simulink model "altit"  (Simulink 5.0)
settings: Solver=ode23  SolverMode=SingleTasking  StartTime=0.0  StopTime=300  RelTol=1e-3  AbsTol=1e-6
values from neighbouring files (symbols this model uses):
  A = [Xu/m Xw/m 0 -g*cos(theta0) 0;[Zu Zw Zq+m*U0 -m*g*sin(theta0)]/(m-Zwd) 0 ... (first row only)    [altit_simul.m]    (also in lecture11.m = [Yv/m Yp/m (Yr/m-U0) g*cos(theta0); lecture4.m = [Xu/m Xw/m 0 -g*cos(theta0);[Zu Zw Zq+m*U0 -m*g*sin(theta0)])
  B = [Xde/m Xdp/m;Zde/(m-Zwd) Zdp/(m-Zwd);(Mde+Zde*Mwd/(m-Zwd))/Iyy    (Mdp+Zdp*Mwd/(m-Zwd))/Iyy;0 0;0 0]    [altit_simul.m]    (also in lecture11.m = [1/m 0 0;0 1/Ixxp Ixzp;0 Ixzp 1/Izzp;0 0 0]*[Yda Ydr;Lda Ldr; lecture4.m = [Xde/m Xdp/m;Zde/(m-Zwd) Zdp/(m-Zwd);(Mde+Zde*Mwd/(m-Zwd))/I)
  C = [eye(5);zeros(2,5)]    [altit_simul.m]    (also in hw7_1_6243_2003.m = [0 1 r]/[x0 B A*x0]; lecture11.m = [eye(4)]; lecture4.m = [eye(4,4);0 -1/U0 0 1])
  D = [zeros(5,2);[eye(2)]]    [altit_simul.m]    (also in lecture11.m = V; lecture4.m = V)
  JDe = [tau_e 1]    [altit_simul.m]
  JDt = [tau_t 1]    [altit_simul.m]
  JNe = 1    [altit_simul.m]
  JNt = 1    [altit_simul.m]
  K_h = -1*.00116    (= -0.00116)    [altit_simul.m]
  K_q = 1.95*K_th    (= 1.95)    [altit_simul.m]
  K_th = 1    [altit_simul.m]
  K_u = .1    (= 0.1)    [altit_simul.m]
  Khd = [1/(8*abs(tt(ii))) 1]    [altit_simul.m]
  Khn = [1/abs(tt(ii)) 1]    [altit_simul.m]
  Kud = [1/(0.2857*5) 1]    [altit_simul.m]
  Kun = [1/0.2857 1]    [altit_simul.m]
undefined symbols (not defined in the file or in its folder): sigbuilder_block
libraries: simulink x1
settings Model: LastModifiedBy=jonathan How  LimitDataPoints=off  BooleanDataType=off

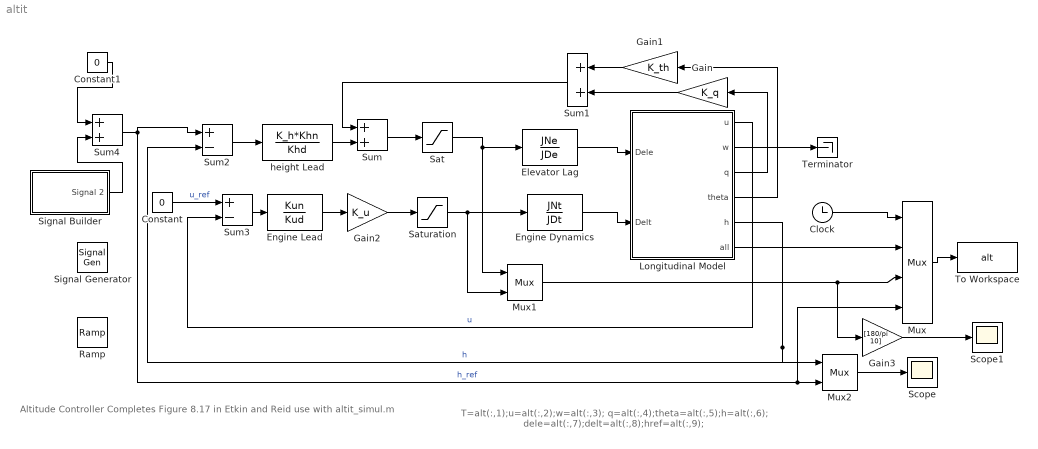
== system altit ==
  note: Altitude Controller
      | Completes Figure 8.17 in Etkin and Reid
      | use with altit_simul.m
  note: T=alt(:,1);u=alt(:,2);w=alt(:,3);
      | q=alt(:,4);theta=alt(:,5);h=alt(:,6);
      | dele=alt(:,7);delt=alt(:,8);href=alt(:,9);
  Clock : Clock
      settings: Decimation=10
  Constant : Constant  Value=0
  Constant1 : Constant  Value=0
  Elevator Lag : TransferFcn  Numerator=JNe  Denominator=JDe
  Engine Dynamics : TransferFcn  Numerator=JNt  Denominator=JDt
  Engine Lead : TransferFcn  Numerator=Kun  Denominator=Kud
  Gain : Gain  Orientation=left  Gain=K_q  SaturateOnIntegerOverflow=on
  Gain1 : Gain  Orientation=left  Gain=K_th  SaturateOnIntegerOverflow=on
  Gain2 : Gain  Gain=K_u  SaturateOnIntegerOverflow=on
  Gain3 : Gain  Gain=[180/pi 10]  SaturateOnIntegerOverflow=on
  Longitudinal Model : Subsystem
  Mux : Mux
  Mux1 : Mux  Inputs=2
  Mux2 : Mux  Inputs=2
  Ramp : simulink/Sources/Ramp  slope=15  start=5  X0=0
  Sat : Saturate  UpperLimit=20*pi/180  LowerLimit=-20*pi/180
  Saturation : Saturate  UpperLimit=.2  LowerLimit=-.219
  Scope : Scope
      settings: TickLabels=on  TimeRange=300  YMin=-200  YMax=1600  DataFormat=Array
  Scope1 : Scope
      settings: TickLabels=on  TimeRange=300  YMax=10  DataFormat=Array
  Signal Generator : SignalGenerator  WaveForm=sawtooth  Amplitude=100  Frequency=1/20
  Signal Builder : Subsystem  Tag=STV Subsys  StartFcn=sigbuilder_block('start');  StopFcn=sigbuilder_block('stop');  ClipboardFcn=sigbuilder_block('clipboard');  mask(Sigbuilder block){}
      mask help: Sigbuilder GUI
      mask init:
      | if ~strcmp(get_param(bdroot(gcb),'SimulationStatus'),'stopped') tuvar = sigbuilder_block('maskInit'); end
      settings: CopyFcn=sigbuilder_block('copy');  DeleteFcn=sigbuilder_block('delete');  ModelCloseFcn=sigbuilder_block('modelClose');  PreSaveFcn=sigbuilder_block('preSave');  NameChangeFcn=sigbuilder_block('namechange');  OpenFcn=sigbuilder_block('open',[50.25 340.5 519.75 399.75 ]);  CloseFcn=sigbuilder_block('close');
      mask Display: plot(0,0,100,100,[10,10,40,40,10],[80,20,20,80,80],[40,10],[50,50], [40,27,10],[65,72,56],[40,25,25,10],[28,28,43,43]);
  Sum : Sum  SaturateOnIntegerOverflow=on  InputSameDT=on
  Sum1 : Sum  Orientation=left  SaturateOnIntegerOverflow=on  InputSameDT=on
  Sum2 : Sum  Inputs=+-  SaturateOnIntegerOverflow=on  InputSameDT=on
  Sum3 : Sum  Inputs=+-  SaturateOnIntegerOverflow=on  InputSameDT=on
  Sum4 : Sum  SaturateOnIntegerOverflow=on  InputSameDT=on
  Terminator : Terminator
  To Workspace : ToWorkspace  VariableName=alt  SampleTime=-1  SaveFormat=Array
  height Lead : TransferFcn  Numerator=K_h*Khn  Denominator=Khd
  wires:
  Elevator Lag/1 -> Longitudinal Model/1(Dele)
  Engine Dynamics/1 -> Longitudinal Model/2(Delt)
  Longitudinal Model/3(q) -> Gain/1
  Longitudinal Model/4(theta) -> Gain1/1
  Gain1/1 -> Sum1/1
  Gain/1 -> Sum1/2
  Sum1/1 -> Sum/1
  Engine Lead/1 -> Gain2/1
  Gain2/1 -> Saturation/1
  Sum2/1 -> height Lead/1
  height Lead/1 -> Sum/2
  Longitudinal Model/6(all) -> Mux/2
  Clock/1 -> Mux/1
  Mux/1 -> To Workspace/1
  Longitudinal Model/1(u) -> Sum3/2  "u"
  Sum3/1 -> Engine Lead/1
  Constant/1 -> Sum3/1  "u_ref"
  Sum/1 -> Sat/1
  Longitudinal Model/2(w) -> Terminator/1
  Sat/1 -> Elevator Lag/1, Mux1/1
  Saturation/1 -> Engine Dynamics/1, Mux1/2
  Mux2/1 -> Scope/1
  Mux1/1 -> Mux/3, Gain3/1
  Constant1/1 -> Sum4/1
  Sum4/1 -> Mux2/2, Mux/4, Sum2/1  "h_ref"
  Longitudinal Model/5(h) -> Mux2/1, Sum2/2  "h"
  Signal Builder/1(Signal 2) -> Sum4/2
  Gain3/1 -> Scope1/1

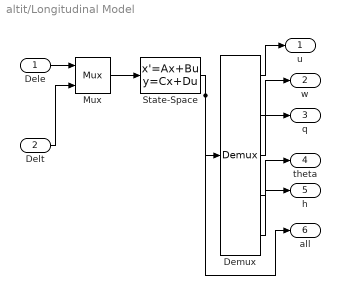
== system altit/Longitudinal Model ==
  Dele : Inport
  Delt : Inport  Port=2
  Demux : Demux  Outputs=5
  Mux : Mux  Inputs=2
  State-Space : StateSpace  A=A  B=B  C=C(1:5,:)  D=D(1:5,:)  X0=[0 0 0 0 0 0 0]
  u : Outport  InitialOutput=0
  w : Outport  Port=2  InitialOutput=0
  q : Outport  Port=3  InitialOutput=0
  theta : Outport  Port=4  InitialOutput=0
  h : Outport  Port=5  InitialOutput=0
  all : Outport  Port=6  InitialOutput=0
  wires:
  Mux/1 -> State-Space/1
  Demux/1 -> u/1
  Dele/1 -> Mux/1
  Demux/2 -> w/1
  Demux/3 -> q/1
  Demux/4 -> theta/1
  Demux/5 -> h/1
  Delt/1 -> Mux/2
  State-Space/1 -> Demux/1, all/1

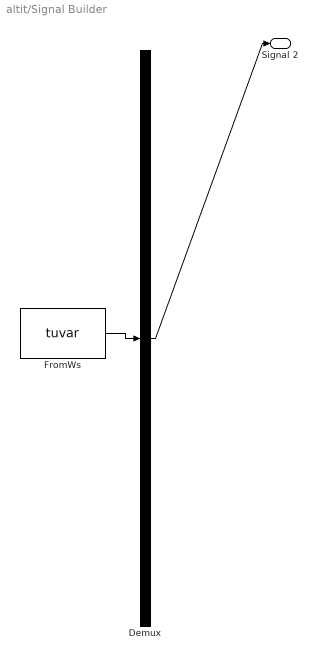
== system altit/Signal Builder ==
  Demux : Demux  Tag=STV Demux  Outputs=1
  FromWs : FromWorkspace  Tag=STV FromWs  VariableName=tuvar  SampleTime=0  SigBuilderData=DataTag0
      SigBuilderData=|
      | channels.label = 'Signal 2'
      | channels.allXData = {[0 25 125 125 175 175 275 300 300]}
      | channels.allYData = {[0 0 1500 1500 1500 1500 0 0 -10]}
      | dataSet.timeRange = [0 300]
      | dataSet.name = 'Group 1'
  Signal 2 : Outport  Tag=STV Outport
  wires:
  FromWs/1 -> Demux/1
  Demux/1 -> Signal 2/1
